simulink model "B2_Parallel_Model"  (Simulink 7.7)
settings: Solver=ode45  StartTime=0.0  StopTime=1650  MaxStep=0.5  RelTol=1e-3
values from neighbouring files (symbols this model uses):
  B_OCV = B_OCV(i)    [B2_Parallel_Model1.m]
  B_SOC = 1-[  0   8  20  40  60    80   90   95    99 100]/100    [B2_Parallel_Model1.m]
libraries: simulink x3
settings Model: Creator=jnaber  LastModifiedBy=Arjun
settings SolverCC: InitialStep=0.01
settings OptimizationCC: InitFltsAndDblsToZero=on
settings DebuggingCC: SaveWithParameterizedLinksMsg=none  StrictBusMsg=Warning
settings GRTTargetCC: TargetFcnLib=ansi_tfl_tmw.mat

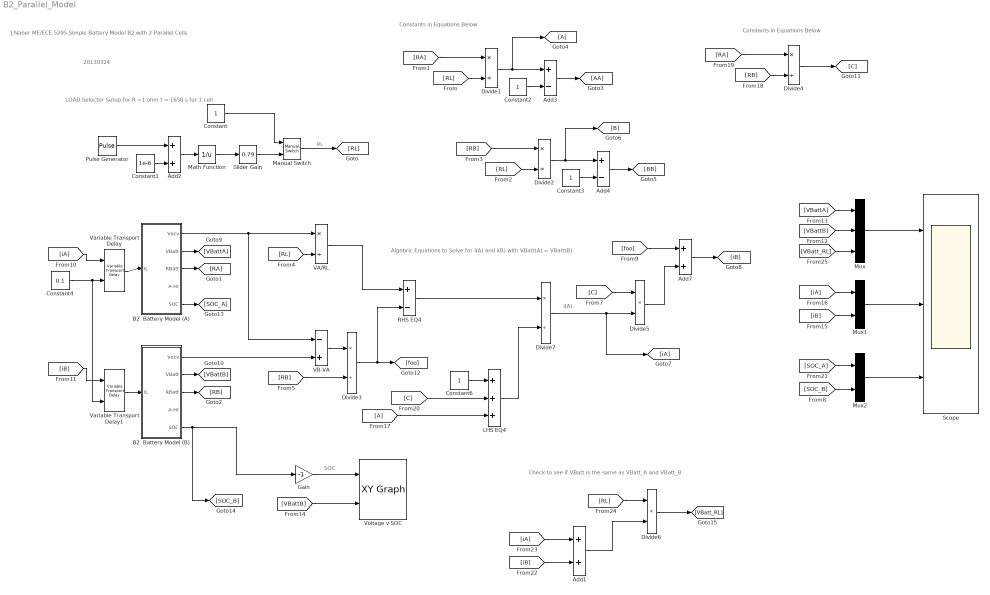
== system B2_Parallel_Model ==
  note: J.Naber
      | ME/ECE 5295
      | Simple Battery Model
      | B2 with 2 Parallel Cells
  note: 20130324
  note: SOC
  note: i(A)
  note: LOAD Selector
      | Setup for R =1 ohm
      | t = 1650 s
      | for 1 cell
  note: Check to see if VBatt is the same as VBatt_A and VBatt_B
  note: Constants in Equations Below
  note: Constants in Equations Below
  note: Algebric Equations to Solve for
      | i(A) and i(B) with VBatt(A) = VBatt(B)
  Add1 : Sum
  Add2 : Sum
  Add3 : Sum  Inputs=+-
  Add4 : Sum  Inputs=+-
  Add7 : Sum
  B2  Battery Model (A) : Subsystem  mask{CAP=1, RBatt=0.01, NCell=1}
      mask prompts: CAP "Capacity Per Cell (Ah)"; RBatt "Battery Resistance Per Cell (Ohm)"; NCell "Number of Cells (-)"
  B2  Battery Model (B) : Subsystem  mask{CAP=0.8, RBatt=0.01, NCell=1}
      mask prompts: CAP "Capacity Per Cell (Ah)"; RBatt "Battery Resistance Per Cell (Ohm)"; NCell "Number of Cells (-)"
  Constant{,2..3,6} (4 alike) : Constant
  Constant1 : Constant  Value=1e-6
  Constant4 : Constant  Value=0.1
  Divide{1..4,7} (5 alike) : Product  Inputs=*/
  Divide5 : Product  Inputs=**
  Divide6 : Product  Inputs=**
  Gain : Gain  Gain=-1
  LHS EQ4 : Sum  Inputs=+++
  Manual Switch : simulink/Signal Routing/Manual Switch  SystemSampleTime=-1  sw=1  action=0  varsize=off
  Math Function : Math  Operator=reciprocal  SaturateOnIntegerOverflow=on
  Mux : Mux  Inputs=3
  Mux1 : Mux  Inputs=2
  Mux2 : Mux  Inputs=2
  Pulse Generator : DiscretePulseGenerator  PulseType=Time based  Period=10  PulseWidth=80  PhaseDelay=5
  RHS EQ4 : Sum  Inputs=+-
  Scope : Scope  NumInputPorts=3
      settings: TimeRange=1800  YMin=2~-0.5~0  YMax=5~3~1  MaxDataPoints=25000  Decimation=2
  Slider Gain : simulink/Math Operations/Slider Gain  SystemSampleTime=-1  low=0  gain=0.79  high=2
  VA/RL : Product  Inputs=*/
  VB-VA : Sum  Inputs=-+
  Variable Transport Delay : VariableTransportDelay  MaximumDelay=10  InitialOutput=1*3.8/1/2
  Variable Transport Delay1 : VariableTransportDelay  MaximumDelay=10  InitialOutput=1*3.8/1/2
  Voltage v SOC : simulink/Sinks/XY Graph  SystemSampleTime=-1  xmin=-1  xmax=0  ymin=0  ymax=4.5  st=-1
  wires:
  Gain/1 -> Voltage v SOC/1
  Constant/1 -> Manual Switch/1
  Slider Gain/1 -> Manual Switch/2
  Pulse Generator/1 -> Add2/1
  Constant1/1 -> Add2/2
  Add2/1 -> Math Function/1
  Math Function/1 -> Slider Gain/1
  Manual Switch/1 -> [RL]  "RL"
  B2  Battery Model (B)/3(RBatt) -> [RB]
  [RL] -> Divide1/2
  [RA] -> Divide1/1
  Divide1/1 -> Add3/1, [A]
  Add3/1 -> [AA]
  Constant2/1 -> Add3/2
  [RL] -> Divide2/2
  [RB] -> Divide2/1
  Divide2/1 -> Add4/1, [B]
  Add4/1 -> [BB]
  Constant3/1 -> Add4/2
  B2  Battery Model (A)/1(Vocv) -> VA/RL/1, VB-VA/1
  [RL] -> VA/RL/2
  B2  Battery Model (B)/1(Vocv) -> VB-VA/2
  Divide7/1 -> [iA], Divide5/2
  [foo] -> Add7/1
  Add7/1 -> [iB]
  B2  Battery Model (A)/2(VBatt) -> [VBattA]
  B2  Battery Model (B)/2(VBatt) -> [VBattB]
  [VBattA] -> Mux/1
  [VBattB] -> Mux/2
  Mux/1 -> Scope/1
  B2  Battery Model (B)/5(SOC) -> Gain/1, [SOC_B]
  [VBattB] -> Voltage v SOC/2
  Variable Transport Delay/1 -> B2  Battery Model (A)/1(IL)
  [iA] -> Variable Transport Delay/1
  Variable Transport Delay1/1 -> B2  Battery Model (B)/1(IL)
  [iB] -> Variable Transport Delay1/1
  [iA] -> Mux1/1
  [iB] -> Mux1/2
  Mux1/1 -> Scope/2
  VB-VA/1 -> Divide3/1
  [RB] -> Divide3/2
  VA/RL/1 -> RHS EQ4/1
  Divide3/1 -> RHS EQ4/2, [foo]
  Constant6/1 -> LHS EQ4/1
  [A] -> LHS EQ4/3
  [RA] -> Divide4/1
  [RB] -> Divide4/2
  Divide4/1 -> [C]
  [C] -> LHS EQ4/2
  RHS EQ4/1 -> Divide7/1
  LHS EQ4/1 -> Divide7/2
  [C] -> Divide5/1
  Divide5/1 -> Add7/2
  [SOC_A] -> Mux2/1
  [SOC_B] -> Mux2/2
  Mux2/1 -> Scope/3
  [iA] -> Add1/1
  [iB] -> Add1/2
  [RL] -> Divide6/1
  Add1/1 -> Divide6/2
  Divide6/1 -> [VBatt_RL]
  [VBatt_RL] -> Mux/3
  B2  Battery Model (A)/5(SOC) -> [SOC_A]
  B2  Battery Model (A)/3(RBatt) -> [RA]
  Constant4/1 -> Variable Transport Delay/2, Variable Transport Delay1/2

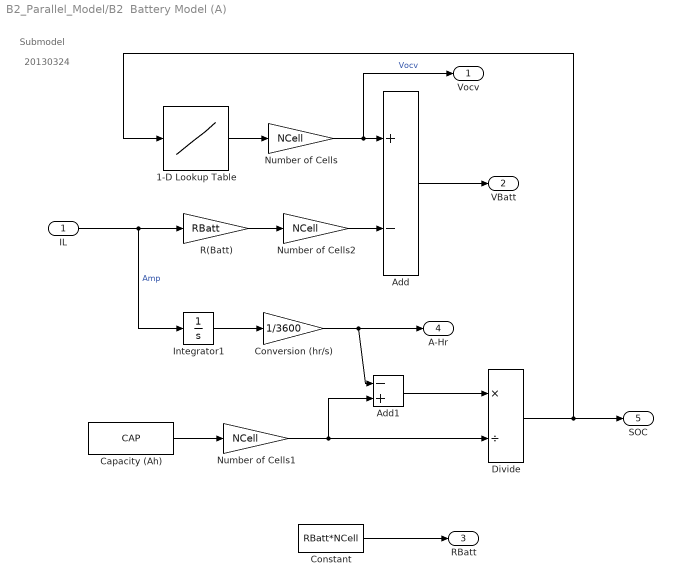
== system B2_Parallel_Model/B2  Battery Model (A) ==
  note: Submodel
  note: 20130324
  IL : Inport
  1-D Lookup Table : Lookup_n-D  NumberOfTableDimensions=1  BreakpointsForDimension1=B_SOC  Table=B_OCV  ExtrapMethod=Clip  UseLastTableValue=on  RndMeth=Simplest  InputSameDT=on
  Add : Sum  Inputs=+-
  Add1 : Sum  Inputs=-+
  Capacity (Ah) : Constant  Value=CAP
  Constant : Constant  Value=RBatt*NCell
  Conversion (hr/s) : Gain  Gain=1/3600
  Divide : Product  Inputs=*/
  Integrator1 : Integrator  InitialCondition=50
  Number of Cells : Gain  Gain=NCell
  Number of Cells1 : Gain  Gain=NCell
  Number of Cells2 : Gain  Gain=NCell
  R(Batt) : Gain  Gain=RBatt
  Vocv : Outport
  VBatt : Outport  Port=2
  RBatt : Outport  Port=3
  A-Hr : Outport  Port=4
  SOC : Outport  Port=5
  wires:
  1-D Lookup Table/1 -> Number of Cells/1
  R(Batt)/1 -> Number of Cells2/1
  Add/1 -> VBatt/1
  Integrator1/1 -> Conversion (hr/s)/1
  IL/1 -> R(Batt)/1, Integrator1/1  "Amp"
  Conversion (hr/s)/1 -> A-Hr/1, Add1/1
  Capacity (Ah)/1 -> Number of Cells1/1
  Add1/1 -> Divide/1
  Divide/1 -> SOC/1, 1-D Lookup Table/1
  Number of Cells/1 -> Add/1, Vocv/1  "Vocv"
  Number of Cells1/1 -> Add1/2, Divide/2
  Number of Cells2/1 -> Add/2
  Constant/1 -> RBatt/1

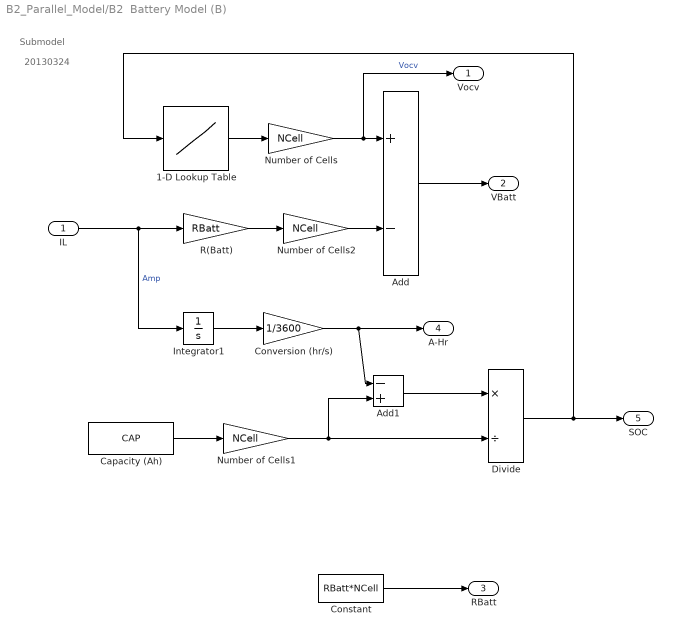
== system B2_Parallel_Model/B2  Battery Model (B) ==
  note: 20130324
  note: Submodel
  IL : Inport
  1-D Lookup Table : Lookup_n-D  NumberOfTableDimensions=1  BreakpointsForDimension1=B_SOC  Table=B_OCV  ExtrapMethod=Clip  UseLastTableValue=on  RndMeth=Simplest  InputSameDT=on
  Add : Sum  Inputs=+-
  Add1 : Sum  Inputs=-+
  Capacity (Ah) : Constant  Value=CAP
  Constant : Constant  Value=RBatt*NCell
  Conversion (hr/s) : Gain  Gain=1/3600
  Divide : Product  Inputs=*/
  Integrator1 : Integrator  InitialCondition=50
  Number of Cells : Gain  Gain=NCell
  Number of Cells1 : Gain  Gain=NCell
  Number of Cells2 : Gain  Gain=NCell
  R(Batt) : Gain  Gain=RBatt
  Vocv : Outport
  VBatt : Outport  Port=2
  RBatt : Outport  Port=3
  A-Hr : Outport  Port=4
  SOC : Outport  Port=5
  wires:
  Number of Cells2/1 -> Add/2
  Number of Cells1/1 -> Divide/2, Add1/2
  Number of Cells/1 -> Vocv/1, Add/1  "Vocv"
  Divide/1 -> 1-D Lookup Table/1, SOC/1
  Add1/1 -> Divide/1
  Capacity (Ah)/1 -> Number of Cells1/1
  Conversion (hr/s)/1 -> Add1/1, A-Hr/1
  IL/1 -> Integrator1/1, R(Batt)/1  "Amp"
  Integrator1/1 -> Conversion (hr/s)/1
  Add/1 -> VBatt/1
  R(Batt)/1 -> Number of Cells2/1
  1-D Lookup Table/1 -> Number of Cells/1
  Constant/1 -> RBatt/1
